simulink model "gm_soc_dvbs2_fpga"  (R2025b)
settings: Solver=VariableStepAuto  StartTime=0.0  StopTime=10.0  RelTol=1e-3
InitFcn:
  | soc_dvbs2_init;
undefined symbols (not defined in the file or in its folder): Add, coefficientsLog, coefficientsSqrt1, coefficientsSqrt2, dataBits, Deinterleaver, designMultirateFIR, noisePow, Shift, Short, soc_dvbs2_designFIRFilter, soc_dvbs2_txPacketBits, syncWord, txDataOut, txFiltCoeff, XData
libraries: simulink x304, hdlsllib x265, dspsigops x15, dsphdlfiltering2 x8, hdlmdlgenlib x6, dsphdlsigops2 x5, commseqgen3 x5, dsphdlmathfun2 x3, hwlogicconnlib x2, whdledac x2, commhdlcrc x2, whdlutilities x1
(part 25 of 36)

== system gm_soc_dvbs2_fpga/DVBS2/DVBS2 TxRx/Channel/AWGN Generator/Unit Variance Gaussian Noise/logImplementation/log/RangeReconstruction ==
  y_e : Inport  OutDataTypeStr=fixdt(1, 31, 27)  PortDimensions=1  SampleTime=6.25e-08
  exp_e : Inport  Port=2  OutDataTypeStr=uint8  PortDimensions=1  SampleTime=6.25e-08
  Add1 : Sum  Inputs=+-  OutDataTypeStr=fixdt(0, 31, 24)  AccumDataTypeStr=fixdt(1, 36, 28)  SampleTime=6.25e-08
  Bit Shift : hdlsllib/Logic and Bit Operations/Bit Shift  mode=Shift Left Logical  N=double(1)
  Constant : Constant  Value=0.69314718060195446014404296875  OutDataTypeStr=fixdt(1, 33, 32)  SampleTime=6.25e-08
  Delay{1..6} (6 alike) : Delay  DelayLength=double(2)  InitialCondition=0  SampleTime=6.25e-08
  Product : Product  Inputs=**  OutDataTypeStr=fixdt(1, 41, 32)  SampleTime=6.25e-08
  Product_out_dtc : DataTypeConversion  OutDataTypeStr=fixdt(1, 35, 28)  SampleTime=6.25e-08  SaturateOnIntegerOverflow=off  RndMeth=Floor
  e : Outport  SampleTime=6.25e-08
  wires:
  Delay1/1 -> Delay5/1
  Delay5/1 -> Add1/2
  y_e/1 -> Delay1/1
  Delay2/1 -> Product/2
  Delay3/1 -> Product/1
  Constant/1 -> Delay2/1
  exp_e/1 -> Delay3/1
  Product_out_dtc/1 -> Delay4/1
  Product/1 -> Product_out_dtc/1
  Delay4/1 -> Add1/1
  Delay6/1 -> Bit Shift/1
  Add1/1 -> Delay6/1
  Bit Shift/1 -> e/1

== system gm_soc_dvbs2_fpga/DVBS2/DVBS2 TxRx/Channel/AWGN Generator/Unit Variance Gaussian Noise/logImplementation/log/RangeReduction ==
  note: Range of x_e=[1,2)
  x : Inport  OutDataTypeStr=fixdt(0, 48, 48)  PortDimensions=1  SampleTime=6.25e-08
  Add : Sum  OutDataTypeStr=fixdt(0,49,48)
  Constant : Constant  OutDataTypeStr=uint8  SampleTime=-1
  Delay : Delay
  Delay{1,3..7} (6 alike) : Delay  DelayLength=1
  Delay2 : Delay
  Shift Arithmetic3 : ArithShift  BitShiftNumberSource=Input port  BitShiftNumber=8  BitShiftDirection=Left
      settings: InputPortMap=u0,p1
  leadingZeroDetector : MATLAB Function  TreatAsAtomicUnit=on
  x_e : Outport  SampleTime=6.25e-08
  exp_e : Outport  Port=2  SampleTime=6.25e-08  VectorParamsAs1DForOutWhenUnconnected=off
  wires:
  x/1 -> Delay3/1, Delay1/1
  leadingZeroDetector/1(exp_e) -> Delay2/1  "exp_e-1"
  Delay5/1 -> Delay7/1
  Delay2/1 -> Shift Arithmetic3/2, Delay5/1
  Delay/1 -> Shift Arithmetic3/1
  Delay3/1 -> Delay/1
  Delay1/1 -> leadingZeroDetector/1(x)
  Shift Arithmetic3/1 -> Delay4/1
  Delay4/1 -> Add/1
  Delay7/1 -> exp_e/1
  Constant/1 -> Add/2
  Add/1 -> Delay6/1
  Delay6/1 -> x_e/1

== system gm_soc_dvbs2_fpga/DVBS2/DVBS2 TxRx/DVB-S2 HDL Receiver/Demod Deinterleave and FECDecode/DVBS2 HDL Deinterleaver/RAM Address Generator/Generate and Add Read Base Address/Indicate End of Every ShortFrame Length Samples ==
  readAddr : Inport  OutDataTypeStr=fixdt(0, 17, 0)  PortDimensions=1  SampleTime=7.8125e-09
  Compare To Constant : simulink/Logic and Bit Operations/Compare To Constant  relop===  const=ConfigRx.ShortFrameLen - 1  OutDataTypeStr=boolean
  Compare To Constant1 : simulink/Logic and Bit Operations/Compare To Constant  relop===  const=ConfigRx.ShortFrameLen*2 - 1  OutDataTypeStr=boolean
  Compare To Constant2 : simulink/Logic and Bit Operations/Compare To Constant  relop===  const=ConfigRx.ShortFrameLen*3 - 1  OutDataTypeStr=boolean
  Compare To Constant3 : simulink/Logic and Bit Operations/Compare To Constant  relop===  const=ConfigRx.ShortFrameLen*4 - 1  OutDataTypeStr=boolean
  Logical Operator1 : Logic  Operator=OR  Inputs=4  AllPortsSameDT=off  OutDataTypeStr=boolean
  endIndicate : Outport  SampleTime=7.8125e-09
  wires:
  Compare To Constant/1 -> Logical Operator1/1
  readAddr/1 -> Compare To Constant3/1, Compare To Constant1/1, Compare To Constant2/1, Compare To Constant/1
  Compare To Constant2/1 -> Logical Operator1/3
  Compare To Constant1/1 -> Logical Operator1/2
  Logical Operator1/1 -> endIndicate/1
  Compare To Constant3/1 -> Logical Operator1/4

== system gm_soc_dvbs2_fpga/DVBS2/DVBS2 TxRx/DVB-S2 HDL Receiver/Demod Deinterleave and FECDecode/DVBS2 HDL Deinterleaver/RAM Address Generator/Read Offset Address/Compute Read Offset Address ==
  curR : Inport  OutDataTypeStr=uint16  PortDimensions=1  SampleTime=7.8125e-09
  maxC : Inport  Port=2  OutDataTypeStr=fixdt(0, 3, 0)  PortDimensions=1  SampleTime=7.8125e-09
  curC : Inport  Port=3  OutDataTypeStr=fixdt(0, 3, 0)  PortDimensions=1  SampleTime=7.8125e-09
  Add : Sum  OutDataTypeStr=fixdt(0, 17, 0)
  Delay1 : Delay  DelayLength=1
  Delay2 : Delay
  Delay3 : Delay
  Delay4 : Delay  DelayLength=1
  Delay5 : Delay  DelayLength=1
  Delay8 : Delay
  Product : Product  OutDataTypeStr=fixdt('ufix17')
  addr : Outport  SampleTime=7.8125e-09
  wires:
  Delay1/1 -> Add/1
  Delay3/1 -> Delay4/1
  Delay2/1 -> Product/2
  Delay5/1 -> addr/1
  maxC/1 -> Delay2/1
  curR/1 -> Delay8/1
  Product/1 -> Delay1/1
  Add/1 -> Delay5/1
  Delay8/1 -> Product/1
  curC/1 -> Delay3/1
  Delay4/1 -> Add/2

== system gm_soc_dvbs2_fpga/DVBS2/DVBS2 TxRx/DVB-S2 HDL Receiver/Demod Deinterleave and FECDecode/DVBS2 HDL Deinterleaver/RAM Address Generator/Read Offset Address/Generate Signal for End of Frame ==
  maxR : Inport  OutDataTypeStr=uint16  PortDimensions=1  SampleTime=7.8125e-09
  maxC : Inport  Port=2  OutDataTypeStr=fixdt(0, 3, 0)  PortDimensions=1  SampleTime=7.8125e-09
  Add : Sum  Inputs=+-  OutDataTypeStr=uint16
  Compare To Constant : simulink/Logic and Bit Operations/Compare To Constant  relop=~=  const=0  OutDataTypeStr=boolean
  Constant : Constant  OutDataTypeStr=fixdt('ufix1')  SampleTime=Tsamp
  Constant1 : Constant  Value=0  OutDataTypeStr=fixdt('ufix1')  SampleTime=Tsamp
  Delay : Delay
  Delay1 : Delay
  Delay2 : Delay  DelayLength=1
  Delay4 : Delay  DelayLength=1
  Product : Product  OutDataTypeStr=uint16
  Switch : Switch  Criteria=u2 > Threshold  OutDataTypeStr=fixdt(0, 1, 0)  SaturateOnIntegerOverflow=off  InputSameDT=off
  chkwrAddrEnd : Outport  SampleTime=7.8125e-09
  wires:
  Constant/1 -> Switch/1
  Delay2/1 -> Add/1, Compare To Constant/1
  Constant1/1 -> Switch/3
  Product/1 -> Delay2/1
  Delay1/1 -> Product/2
  maxR/1 -> Delay/1
  Delay/1 -> Product/1
  maxC/1 -> Delay1/1
  Switch/1 -> Add/2
  Compare To Constant/1 -> Switch/2
  Delay4/1 -> chkwrAddrEnd/1
  Add/1 -> Delay4/1

== system gm_soc_dvbs2_fpga/DVBS2/DVBS2 TxRx/DVB-S2 HDL Receiver/Demod Deinterleave and FECDecode/DVBS2 HDL Deinterleaver/RAM Address Generator/Read Offset Address/Read Offset Address Signals Generator ==
  maxR : Inport  OutDataTypeStr=uint16  PortDimensions=1  SampleTime=7.8125e-09
  chkwrAddrEnd : Inport  Port=2  OutDataTypeStr=uint16  PortDimensions=1  SampleTime=7.8125e-09
  maxC : Inport  Port=3  OutDataTypeStr=fixdt(0, 3, 0)  PortDimensions=1  SampleTime=7.8125e-09
  modcodIs12 : Inport  Port=4  OutDataTypeStr=boolean  PortDimensions=1  SampleTime=7.8125e-09
  wrAddr : Inport  Port=5  OutDataTypeStr=uint16  PortDimensions=1  SampleTime=7.8125e-09
  wrEnb : Inport  Port=6  OutDataTypeStr=boolean  PortDimensions=1  SampleTime=7.8125e-09
  Read Offset Address Signals Generator : MATLAB Function  TreatAsAtomicUnit=on  mask{isInterleave=0}
  Read Offset Address Signals Generator_term3 : Terminator
  t : Constant  Value=double(0)  OutDataTypeStr=boolean  SampleTime=7.8125e-09
  curCorROut : Outport  SampleTime=7.8125e-09  VectorParamsAs1DForOutWhenUnconnected=off
  maxRorCOut : Outport  Port=2  SampleTime=7.8125e-09
  curRorCOut : Outport  Port=3  SampleTime=7.8125e-09
  modcodIs12Out : Outport  Port=4  SampleTime=7.8125e-09
  startOut : Outport  Port=5  SampleTime=7.8125e-09
  endOut : Outport  Port=6  SampleTime=7.8125e-09
  readValid : Outport  Port=7  SampleTime=7.8125e-09
  wires:
  t/1 -> modcodIs12Out/1
  maxR/1 -> Read Offset Address Signals Generator/1(maxR)
  wrEnb/1 -> Read Offset Address Signals Generator/6(wrEnb)
  modcodIs12/1 -> Read Offset Address Signals Generator/4(modcodIs12)
  maxC/1 -> Read Offset Address Signals Generator/3(maxC)
  chkwrAddrEnd/1 -> Read Offset Address Signals Generator/2(chkwrAddrEnd)
  wrAddr/1 -> Read Offset Address Signals Generator/5(wrAddr)
  Read Offset Address Signals Generator/1(curCorROut) -> curCorROut/1
  Read Offset Address Signals Generator/2(maxRorCOut) -> maxRorCOut/1
  Read Offset Address Signals Generator/3(curRorCOut) -> curRorCOut/1
  Read Offset Address Signals Generator/4(modcodIs12Out) -> Read Offset Address Signals Generator_term3/1
  Read Offset Address Signals Generator/5(startOut) -> startOut/1
  Read Offset Address Signals Generator/6(endOut) -> endOut/1
  Read Offset Address Signals Generator/7(readValid) -> readValid/1

== system gm_soc_dvbs2_fpga/DVBS2/DVBS2 TxRx/DVB-S2 HDL Receiver/Stream Recovery/BB Decoder/Extract Stream/Extract User Packet /Indicate SYNCD bit ==
  rst : Inport  OutDataTypeStr=boolean  PortDimensions=1  SampleTime=7.8125e-09
  Distance : Inport  Port=2  OutDataTypeStr=uint16  PortDimensions=1  SampleTime=7.8125e-09
  validIn : Inport  Port=3  OutDataTypeStr=boolean  PortDimensions=1  SampleTime=7.8125e-09
  Constant1 : Constant  OutDataTypeStr=fixdt(0,1,0)  SampleTime=-1
  Constant2 : Constant  Value=0  OutDataTypeStr=fixdt(0,1,0)  SampleTime=-1
  HDL Counter1 : hdlsllib/Sources/HDL Counter  CountType=Free running  CountInit=0  CountStep=1  CountMax=25  CountFromType=Initial value  CountFrom=0  CountResetPort=on  CountLoadPort=off  CountEnbPort=on  CountDirPort=off  CountHitOutputPort=off  CountDataType=Unsigned  CountWordLen=16  CountFracLen=0  CountSampTime=1
  Logical Operator3 : Logic  AllPortsSameDT=off  OutDataTypeStr=boolean
  Relational Operator1 : RelationalOperator  Operator===  OutDataTypeStr=boolean  RndMeth=Simplest  InputSameDT=off
  Subtract1 : Sum  Inputs=+-  OutDataTypeStr=uint16
  Switch : Switch  Criteria=u2 ~= 0  OutDataTypeStr=fixdt(0, 1, 0)  SaturateOnIntegerOverflow=off  InputSameDT=off
  trigger : Outport  SampleTime=7.8125e-09
  wires:
  HDL Counter1/1 -> Relational Operator1/2
  validIn/1 -> HDL Counter1/2, Logical Operator3/2
  rst/1 -> HDL Counter1/1
  Constant2/1 -> Switch/3
  Constant1/1 -> Switch/1
  Distance/1 -> Subtract1/1, Switch/2
  Switch/1 -> Subtract1/2
  Subtract1/1 -> Relational Operator1/1
  Relational Operator1/1 -> Logical Operator3/1
  Logical Operator3/1 -> trigger/1

== system gm_soc_dvbs2_fpga/DVBS2/DVBS2 TxRx/DVB-S2 HDL Receiver/Stream Recovery/BB Decoder/Extract Stream/Extract User Packet /Sample Discard Control ==
  dataIn : Inport  OutDataTypeStr=boolean  PortDimensions=[2]  SampleTime=7.8125e-09
  startIn : Inport  Port=2  OutDataTypeStr=boolean  PortDimensions=1  SampleTime=7.8125e-09
  endIn : Inport  Port=3  OutDataTypeStr=boolean  PortDimensions=1  SampleTime=7.8125e-09
  validIn : Inport  Port=4  OutDataTypeStr=boolean  PortDimensions=1  SampleTime=7.8125e-09
  Sample Discard Control : MATLAB Function  TreatAsAtomicUnit=on
  Sample Discard Control_term1 : Terminator
  t : Constant  Value=double(0)  OutDataTypeStr=boolean  SampleTime=7.8125e-09
  dataOut : Outport  SampleTime=7.8125e-09
  startOut : Outport  Port=2  SampleTime=7.8125e-09
  endOut : Outport  Port=3  SampleTime=7.8125e-09
  validOut : Outport  Port=4  SampleTime=7.8125e-09
  wires:
  t/1 -> startOut/1
  endIn/1 -> Sample Discard Control/3(endIn)
  dataIn/1 -> Sample Discard Control/1(dataIn)
  validIn/1 -> Sample Discard Control/4(validIn)
  startIn/1 -> Sample Discard Control/2(startIn)
  Sample Discard Control/3(endOut) -> endOut/1
  Sample Discard Control/1(dataOut) -> dataOut/1
  Sample Discard Control/2(startOut) -> Sample Discard Control_term1/1
  Sample Discard Control/4(validOut) -> validOut/1

== system gm_soc_dvbs2_fpga/DVBS2/DVBS2 TxRx/DVB-S2 HDL Receiver/Stream Recovery/BB Decoder/Extract Stream/Extract User Packet /Variable Count Limited HDL Counter ==
  rst : Inport  OutDataTypeStr=boolean  PortDimensions=1  SampleTime=7.8125e-09
  countToValue : Inport  Port=2  OutDataTypeStr=uint16  PortDimensions=1  SampleTime=7.8125e-09
  enb : Inport  Port=3  OutDataTypeStr=boolean  PortDimensions=1  SampleTime=7.8125e-09
  Variable Count Limited HDL Counter : MATLAB Function  TreatAsAtomicUnit=on
  Hit : Outport  SampleTime=7.8125e-09
  wires:
  enb/1 -> Variable Count Limited HDL Counter/3(enb)
  rst/1 -> Variable Count Limited HDL Counter/1(rst)
  countToValue/1 -> Variable Count Limited HDL Counter/2(countToValue)
  Variable Count Limited HDL Counter/1(Hit) -> Hit/1

== system gm_soc_dvbs2_fpga/DVBS2/DVBS2 TxRx/DVB-S2 HDL Receiver/Synchronizer and PL Header Decoder/PL Header Recovery/PL Header Decoder/ML Decoder/Compute Euclidean Distance ==
  softBit : Inport  OutDataTypeStr=fixdt(1, 18, 13)  PortDimensions=1  SampleTime=2.5e-07
  Add : Subsystem
  Add1 : Sum  Inputs=+++  OutDataTypeStr=fixdt(1, 20, 13)
  Constant : Constant  OutDataTypeStr=fixdt(0,1,0)  SampleTime=-1
  Data Type Conversion : DataTypeConversion  OutDataTypeStr=fixdt(1, 20, 13)  SaturateOnIntegerOverflow=off  RndMeth=Floor
  Delay{1..7} (7 alike) : Delay
  Divide by 2 : DataTypeConversion  OutDataTypeStr=fixdt(1,18,12)  ConvertRealWorld=Stored Integer (SI)  SaturateOnIntegerOverflow=off  RndMeth=Floor
  Product : Product  OutDataTypeStr=fixdt(1, 18, 13)
  forBit0 : Outport  SampleTime=2.5e-07
  forBit1 : Outport  Port=2  SampleTime=2.5e-07
  wires:
  Delay3/1 -> Add1/3, Add/1(In1)
  Delay5/1 -> Delay6/1
  Delay1/1 -> Product/1
  softBit/1 -> Delay2/1, Delay1/1, Divide by 2/1
  Delay4/1 -> Delay7/1
  Delay2/1 -> Product/2
  Divide by 2/1 -> Delay5/1, Delay4/1
  Product/1 -> Delay3/1
  Constant/1 -> Add1/1, Add/3(In3)
  Delay7/1 -> Add/2(In2)
  Delay6/1 -> Add1/2
  Add/1(Out1) -> Data Type Conversion/1
  Add1/1 -> forBit0/1
  Data Type Conversion/1 -> forBit1/1

== system gm_soc_dvbs2_fpga/DVBS2/DVBS2 TxRx/DVB-S2 HDL Receiver/Synchronizer and PL Header Decoder/PL Header Recovery/PL Header Decoder/ML Decoder/Euclidean Distance Sum Up_instance1 ==
  note: For Each
  Ed0 : Inport  OutDataTypeStr=fixdt(1, 25, 15)  PortDimensions=1  SampleTime=2.5e-07
  Ed1 : Inport  Port=2  OutDataTypeStr=fixdt(1, 20, 13)  PortDimensions=1  SampleTime=2.5e-07
  reset : Inport  Port=3  OutDataTypeStr=boolean  PortDimensions=1  SampleTime=2.5e-07
  CWswitch : Inport  Port=4  OutDataTypeStr=fixdt(0, 1, 0)  PortDimensions=1  SampleTime=2.5e-07
  validIn : Inport  Port=5  OutDataTypeStr=boolean  PortDimensions=1  SampleTime=2.5e-07
  Add : Sum  OutDataTypeStr=fixdt(1, 25, 15)  AccumDataTypeStr=fixdt(1, 26, 15)  SampleTime=2.5e-07
  Delay{1..4} (4 alike) : Delay  DelayLength=double(1)  InitialCondition=0  SampleTime=2.5e-07
  Switch : Switch  Criteria=u2 ~= 0  Threshold="fi(0,0,1,0,\"hex\",\"0\")"  OutDataTypeStr=fixdt(1, 25, 15)  SampleTime=2.5e-07  SaturateOnIntegerOverflow=off  InputSameDT=off
  Unit Delay Enabled Resettable Synchronous : hdlsllib/Discrete/Unit Delay Enabled Resettable Synchronous  InitialCondition=double(0)  SampleTime=-1
  CwEdMetric : Outport  SampleTime=2.5e-07
  wires:
  Ed0/1 -> Switch/3
  reset/1 -> Delay2/1
  validIn/1 -> Delay1/1
  CWswitch/1 -> Switch/2
  Ed1/1 -> Switch/1
  Switch/1 -> Delay3/1
  Delay1/1 -> Unit Delay Enabled Resettable Synchronous/2
  Delay2/1 -> Unit Delay Enabled Resettable Synchronous/3
  Unit Delay Enabled Resettable Synchronous/1 -> Delay4/1, Add/1
  Delay3/1 -> Add/2
  Delay4/1 -> CwEdMetric/1
  Add/1 -> Unit Delay Enabled Resettable Synchronous/1

== system gm_soc_dvbs2_fpga/DVBS2/DVBS2 TxRx/DVB-S2 HDL Receiver/Synchronizer and PL Header Decoder/PL Header Recovery/PL Header Decoder/ML Decoder/Euclidean Distance Sum Up_instance10 ==
  note: For Each
  Ed0 : Inport  OutDataTypeStr=fixdt(1, 25, 15)  PortDimensions=1  SampleTime=2.5e-07
  Ed1 : Inport  Port=2  OutDataTypeStr=fixdt(1, 20, 13)  PortDimensions=1  SampleTime=2.5e-07
  reset : Inport  Port=3  OutDataTypeStr=boolean  PortDimensions=1  SampleTime=2.5e-07
  CWswitch : Inport  Port=4  OutDataTypeStr=fixdt(0, 1, 0)  PortDimensions=1  SampleTime=2.5e-07
  validIn : Inport  Port=5  OutDataTypeStr=boolean  PortDimensions=1  SampleTime=2.5e-07
  Add : Sum  OutDataTypeStr=fixdt(1, 25, 15)  AccumDataTypeStr=fixdt(1, 26, 15)  SampleTime=2.5e-07
  Delay{1..4} (4 alike) : Delay  DelayLength=double(1)  InitialCondition=0  SampleTime=2.5e-07
  Switch : Switch  Criteria=u2 ~= 0  Threshold="fi(0,0,1,0,\"hex\",\"0\")"  OutDataTypeStr=fixdt(1, 25, 15)  SampleTime=2.5e-07  SaturateOnIntegerOverflow=off  InputSameDT=off
  Unit Delay Enabled Resettable Synchronous : hdlsllib/Discrete/Unit Delay Enabled Resettable Synchronous  InitialCondition=double(0)  SampleTime=-1
  CwEdMetric : Outport  SampleTime=2.5e-07
  wires:
  Switch/1 -> Delay3/1
  validIn/1 -> Delay1/1
  Delay1/1 -> Unit Delay Enabled Resettable Synchronous/2
  reset/1 -> Delay2/1
  Delay2/1 -> Unit Delay Enabled Resettable Synchronous/3
  CWswitch/1 -> Switch/2
  Ed1/1 -> Switch/1
  Ed0/1 -> Switch/3
  Unit Delay Enabled Resettable Synchronous/1 -> Delay4/1, Add/1
  Add/1 -> Unit Delay Enabled Resettable Synchronous/1
  Delay3/1 -> Add/2
  Delay4/1 -> CwEdMetric/1

== system gm_soc_dvbs2_fpga/DVBS2/DVBS2 TxRx/DVB-S2 HDL Receiver/Synchronizer and PL Header Decoder/PL Header Recovery/PL Header Decoder/ML Decoder/Euclidean Distance Sum Up_instance11 ==
  note: For Each
  Ed0 : Inport  OutDataTypeStr=fixdt(1, 25, 15)  PortDimensions=1  SampleTime=2.5e-07
  Ed1 : Inport  Port=2  OutDataTypeStr=fixdt(1, 20, 13)  PortDimensions=1  SampleTime=2.5e-07
  reset : Inport  Port=3  OutDataTypeStr=boolean  PortDimensions=1  SampleTime=2.5e-07
  CWswitch : Inport  Port=4  OutDataTypeStr=fixdt(0, 1, 0)  PortDimensions=1  SampleTime=2.5e-07
  validIn : Inport  Port=5  OutDataTypeStr=boolean  PortDimensions=1  SampleTime=2.5e-07
  Add : Sum  OutDataTypeStr=fixdt(1, 25, 15)  AccumDataTypeStr=fixdt(1, 26, 15)  SampleTime=2.5e-07
  Delay{1..4} (4 alike) : Delay  DelayLength=double(1)  InitialCondition=0  SampleTime=2.5e-07
  Switch : Switch  Criteria=u2 ~= 0  Threshold="fi(0,0,1,0,\"hex\",\"0\")"  OutDataTypeStr=fixdt(1, 25, 15)  SampleTime=2.5e-07  SaturateOnIntegerOverflow=off  InputSameDT=off
  Unit Delay Enabled Resettable Synchronous : hdlsllib/Discrete/Unit Delay Enabled Resettable Synchronous  InitialCondition=double(0)  SampleTime=-1
  CwEdMetric : Outport  SampleTime=2.5e-07
  wires:
  Ed0/1 -> Switch/3
  reset/1 -> Delay2/1
  validIn/1 -> Delay1/1
  CWswitch/1 -> Switch/2
  Ed1/1 -> Switch/1
  Switch/1 -> Delay3/1
  Delay1/1 -> Unit Delay Enabled Resettable Synchronous/2
  Delay2/1 -> Unit Delay Enabled Resettable Synchronous/3
  Unit Delay Enabled Resettable Synchronous/1 -> Delay4/1, Add/1
  Add/1 -> Unit Delay Enabled Resettable Synchronous/1
  Delay3/1 -> Add/2
  Delay4/1 -> CwEdMetric/1

== system gm_soc_dvbs2_fpga/DVBS2/DVBS2 TxRx/DVB-S2 HDL Receiver/Synchronizer and PL Header Decoder/PL Header Recovery/PL Header Decoder/ML Decoder/Euclidean Distance Sum Up_instance12 ==
  note: For Each
  Ed0 : Inport  OutDataTypeStr=fixdt(1, 25, 15)  PortDimensions=1  SampleTime=2.5e-07
  Ed1 : Inport  Port=2  OutDataTypeStr=fixdt(1, 20, 13)  PortDimensions=1  SampleTime=2.5e-07
  reset : Inport  Port=3  OutDataTypeStr=boolean  PortDimensions=1  SampleTime=2.5e-07
  CWswitch : Inport  Port=4  OutDataTypeStr=fixdt(0, 1, 0)  PortDimensions=1  SampleTime=2.5e-07
  validIn : Inport  Port=5  OutDataTypeStr=boolean  PortDimensions=1  SampleTime=2.5e-07
  Add : Sum  OutDataTypeStr=fixdt(1, 25, 15)  AccumDataTypeStr=fixdt(1, 26, 15)  SampleTime=2.5e-07
  Delay{1..4} (4 alike) : Delay  DelayLength=double(1)  InitialCondition=0  SampleTime=2.5e-07
  Switch : Switch  Criteria=u2 ~= 0  Threshold="fi(0,0,1,0,\"hex\",\"0\")"  OutDataTypeStr=fixdt(1, 25, 15)  SampleTime=2.5e-07  SaturateOnIntegerOverflow=off  InputSameDT=off
  Unit Delay Enabled Resettable Synchronous : hdlsllib/Discrete/Unit Delay Enabled Resettable Synchronous  InitialCondition=double(0)  SampleTime=-1
  CwEdMetric : Outport  SampleTime=2.5e-07
  wires:
  Switch/1 -> Delay3/1
  validIn/1 -> Delay1/1
  Delay1/1 -> Unit Delay Enabled Resettable Synchronous/2
  reset/1 -> Delay2/1
  Delay2/1 -> Unit Delay Enabled Resettable Synchronous/3
  CWswitch/1 -> Switch/2
  Ed1/1 -> Switch/1
  Ed0/1 -> Switch/3
  Unit Delay Enabled Resettable Synchronous/1 -> Delay4/1, Add/1
  Add/1 -> Unit Delay Enabled Resettable Synchronous/1
  Delay3/1 -> Add/2
  Delay4/1 -> CwEdMetric/1

== system gm_soc_dvbs2_fpga/DVBS2/DVBS2 TxRx/DVB-S2 HDL Receiver/Synchronizer and PL Header Decoder/PL Header Recovery/PL Header Decoder/ML Decoder/Euclidean Distance Sum Up_instance13 ==
  note: For Each
  Ed0 : Inport  OutDataTypeStr=fixdt(1, 25, 15)  PortDimensions=1  SampleTime=2.5e-07
  Ed1 : Inport  Port=2  OutDataTypeStr=fixdt(1, 20, 13)  PortDimensions=1  SampleTime=2.5e-07
  reset : Inport  Port=3  OutDataTypeStr=boolean  PortDimensions=1  SampleTime=2.5e-07
  CWswitch : Inport  Port=4  OutDataTypeStr=fixdt(0, 1, 0)  PortDimensions=1  SampleTime=2.5e-07
  validIn : Inport  Port=5  OutDataTypeStr=boolean  PortDimensions=1  SampleTime=2.5e-07
  Add : Sum  OutDataTypeStr=fixdt(1, 25, 15)  AccumDataTypeStr=fixdt(1, 26, 15)  SampleTime=2.5e-07
  Delay{1..4} (4 alike) : Delay  DelayLength=double(1)  InitialCondition=0  SampleTime=2.5e-07
  Switch : Switch  Criteria=u2 ~= 0  Threshold="fi(0,0,1,0,\"hex\",\"0\")"  OutDataTypeStr=fixdt(1, 25, 15)  SampleTime=2.5e-07  SaturateOnIntegerOverflow=off  InputSameDT=off
  Unit Delay Enabled Resettable Synchronous : hdlsllib/Discrete/Unit Delay Enabled Resettable Synchronous  InitialCondition=double(0)  SampleTime=-1
  CwEdMetric : Outport  SampleTime=2.5e-07
  wires:
  Ed0/1 -> Switch/3
  reset/1 -> Delay2/1
  validIn/1 -> Delay1/1
  CWswitch/1 -> Switch/2
  Ed1/1 -> Switch/1
  Switch/1 -> Delay3/1
  Delay1/1 -> Unit Delay Enabled Resettable Synchronous/2
  Delay2/1 -> Unit Delay Enabled Resettable Synchronous/3
  Unit Delay Enabled Resettable Synchronous/1 -> Delay4/1, Add/1
  Add/1 -> Unit Delay Enabled Resettable Synchronous/1
  Delay3/1 -> Add/2
  Delay4/1 -> CwEdMetric/1

== system gm_soc_dvbs2_fpga/DVBS2/DVBS2 TxRx/DVB-S2 HDL Receiver/Synchronizer and PL Header Decoder/PL Header Recovery/PL Header Decoder/ML Decoder/Euclidean Distance Sum Up_instance14 ==
  note: For Each
  Ed0 : Inport  OutDataTypeStr=fixdt(1, 25, 15)  PortDimensions=1  SampleTime=2.5e-07
  Ed1 : Inport  Port=2  OutDataTypeStr=fixdt(1, 20, 13)  PortDimensions=1  SampleTime=2.5e-07
  reset : Inport  Port=3  OutDataTypeStr=boolean  PortDimensions=1  SampleTime=2.5e-07
  CWswitch : Inport  Port=4  OutDataTypeStr=fixdt(0, 1, 0)  PortDimensions=1  SampleTime=2.5e-07
  validIn : Inport  Port=5  OutDataTypeStr=boolean  PortDimensions=1  SampleTime=2.5e-07
  Add : Sum  OutDataTypeStr=fixdt(1, 25, 15)  AccumDataTypeStr=fixdt(1, 26, 15)  SampleTime=2.5e-07
  Delay{1..4} (4 alike) : Delay  DelayLength=double(1)  InitialCondition=0  SampleTime=2.5e-07
  Switch : Switch  Criteria=u2 ~= 0  Threshold="fi(0,0,1,0,\"hex\",\"0\")"  OutDataTypeStr=fixdt(1, 25, 15)  SampleTime=2.5e-07  SaturateOnIntegerOverflow=off  InputSameDT=off
  Unit Delay Enabled Resettable Synchronous : hdlsllib/Discrete/Unit Delay Enabled Resettable Synchronous  InitialCondition=double(0)  SampleTime=-1
  CwEdMetric : Outport  SampleTime=2.5e-07
  wires:
  Switch/1 -> Delay3/1
  validIn/1 -> Delay1/1
  Delay1/1 -> Unit Delay Enabled Resettable Synchronous/2
  reset/1 -> Delay2/1
  Ed1/1 -> Switch/1
  Delay2/1 -> Unit Delay Enabled Resettable Synchronous/3
  CWswitch/1 -> Switch/2
  Ed0/1 -> Switch/3
  Unit Delay Enabled Resettable Synchronous/1 -> Delay4/1, Add/1
  Add/1 -> Unit Delay Enabled Resettable Synchronous/1
  Delay3/1 -> Add/2
  Delay4/1 -> CwEdMetric/1

== system gm_soc_dvbs2_fpga/DVBS2/DVBS2 TxRx/DVB-S2 HDL Receiver/Synchronizer and PL Header Decoder/PL Header Recovery/PL Header Decoder/ML Decoder/Euclidean Distance Sum Up_instance15 ==
  note: For Each
  Ed0 : Inport  OutDataTypeStr=fixdt(1, 25, 15)  PortDimensions=1  SampleTime=2.5e-07
  Ed1 : Inport  Port=2  OutDataTypeStr=fixdt(1, 20, 13)  PortDimensions=1  SampleTime=2.5e-07
  reset : Inport  Port=3  OutDataTypeStr=boolean  PortDimensions=1  SampleTime=2.5e-07
  CWswitch : Inport  Port=4  OutDataTypeStr=fixdt(0, 1, 0)  PortDimensions=1  SampleTime=2.5e-07
  validIn : Inport  Port=5  OutDataTypeStr=boolean  PortDimensions=1  SampleTime=2.5e-07
  Add : Sum  OutDataTypeStr=fixdt(1, 25, 15)  AccumDataTypeStr=fixdt(1, 26, 15)  SampleTime=2.5e-07
  Delay{1..4} (4 alike) : Delay  DelayLength=double(1)  InitialCondition=0  SampleTime=2.5e-07
  Switch : Switch  Criteria=u2 ~= 0  Threshold="fi(0,0,1,0,\"hex\",\"0\")"  OutDataTypeStr=fixdt(1, 25, 15)  SampleTime=2.5e-07  SaturateOnIntegerOverflow=off  InputSameDT=off
  Unit Delay Enabled Resettable Synchronous : hdlsllib/Discrete/Unit Delay Enabled Resettable Synchronous  InitialCondition=double(0)  SampleTime=-1
  CwEdMetric : Outport  SampleTime=2.5e-07
  wires:
  Ed0/1 -> Switch/3
  reset/1 -> Delay2/1
  validIn/1 -> Delay1/1
  CWswitch/1 -> Switch/2
  Ed1/1 -> Switch/1
  Switch/1 -> Delay3/1
  Delay1/1 -> Unit Delay Enabled Resettable Synchronous/2
  Delay2/1 -> Unit Delay Enabled Resettable Synchronous/3
  Unit Delay Enabled Resettable Synchronous/1 -> Delay4/1, Add/1
  Delay3/1 -> Add/2
  Delay4/1 -> CwEdMetric/1
  Add/1 -> Unit Delay Enabled Resettable Synchronous/1

== system gm_soc_dvbs2_fpga/DVBS2/DVBS2 TxRx/DVB-S2 HDL Receiver/Synchronizer and PL Header Decoder/PL Header Recovery/PL Header Decoder/ML Decoder/Euclidean Distance Sum Up_instance16 ==
  note: For Each
  Ed0 : Inport  OutDataTypeStr=fixdt(1, 25, 15)  PortDimensions=1  SampleTime=2.5e-07
  Ed1 : Inport  Port=2  OutDataTypeStr=fixdt(1, 20, 13)  PortDimensions=1  SampleTime=2.5e-07
  reset : Inport  Port=3  OutDataTypeStr=boolean  PortDimensions=1  SampleTime=2.5e-07
  CWswitch : Inport  Port=4  OutDataTypeStr=fixdt(0, 1, 0)  PortDimensions=1  SampleTime=2.5e-07
  validIn : Inport  Port=5  OutDataTypeStr=boolean  PortDimensions=1  SampleTime=2.5e-07
  Add : Sum  OutDataTypeStr=fixdt(1, 25, 15)  AccumDataTypeStr=fixdt(1, 26, 15)  SampleTime=2.5e-07
  Delay{1..4} (4 alike) : Delay  DelayLength=double(1)  InitialCondition=0  SampleTime=2.5e-07
  Switch : Switch  Criteria=u2 ~= 0  Threshold="fi(0,0,1,0,\"hex\",\"0\")"  OutDataTypeStr=fixdt(1, 25, 15)  SampleTime=2.5e-07  SaturateOnIntegerOverflow=off  InputSameDT=off
  Unit Delay Enabled Resettable Synchronous : hdlsllib/Discrete/Unit Delay Enabled Resettable Synchronous  InitialCondition=double(0)  SampleTime=-1
  CwEdMetric : Outport  SampleTime=2.5e-07
  wires:
  Switch/1 -> Delay3/1
  validIn/1 -> Delay1/1
  Delay1/1 -> Unit Delay Enabled Resettable Synchronous/2
  Ed0/1 -> Switch/3
  reset/1 -> Delay2/1
  Ed1/1 -> Switch/1
  Delay2/1 -> Unit Delay Enabled Resettable Synchronous/3
  CWswitch/1 -> Switch/2
  Unit Delay Enabled Resettable Synchronous/1 -> Add/1, Delay4/1
  Add/1 -> Unit Delay Enabled Resettable Synchronous/1
  Delay3/1 -> Add/2
  Delay4/1 -> CwEdMetric/1

== system gm_soc_dvbs2_fpga/DVBS2/DVBS2 TxRx/DVB-S2 HDL Receiver/Synchronizer and PL Header Decoder/PL Header Recovery/PL Header Decoder/ML Decoder/Euclidean Distance Sum Up_instance17 ==
  note: For Each
  Ed0 : Inport  OutDataTypeStr=fixdt(1, 25, 15)  PortDimensions=1  SampleTime=2.5e-07
  Ed1 : Inport  Port=2  OutDataTypeStr=fixdt(1, 20, 13)  PortDimensions=1  SampleTime=2.5e-07
  reset : Inport  Port=3  OutDataTypeStr=boolean  PortDimensions=1  SampleTime=2.5e-07
  CWswitch : Inport  Port=4  OutDataTypeStr=fixdt(0, 1, 0)  PortDimensions=1  SampleTime=2.5e-07
  validIn : Inport  Port=5  OutDataTypeStr=boolean  PortDimensions=1  SampleTime=2.5e-07
  Add : Sum  OutDataTypeStr=fixdt(1, 25, 15)  AccumDataTypeStr=fixdt(1, 26, 15)  SampleTime=2.5e-07
  Delay{1..4} (4 alike) : Delay  DelayLength=double(1)  InitialCondition=0  SampleTime=2.5e-07
  Switch : Switch  Criteria=u2 ~= 0  Threshold="fi(0,0,1,0,\"hex\",\"0\")"  OutDataTypeStr=fixdt(1, 25, 15)  SampleTime=2.5e-07  SaturateOnIntegerOverflow=off  InputSameDT=off
  Unit Delay Enabled Resettable Synchronous : hdlsllib/Discrete/Unit Delay Enabled Resettable Synchronous  InitialCondition=double(0)  SampleTime=-1
  CwEdMetric : Outport  SampleTime=2.5e-07
  wires:
  Ed0/1 -> Switch/3
  reset/1 -> Delay2/1
  validIn/1 -> Delay1/1
  Delay2/1 -> Unit Delay Enabled Resettable Synchronous/3
  CWswitch/1 -> Switch/2
  Ed1/1 -> Switch/1
  Switch/1 -> Delay3/1
  Delay1/1 -> Unit Delay Enabled Resettable Synchronous/2
  Unit Delay Enabled Resettable Synchronous/1 -> Delay4/1, Add/1
  Delay3/1 -> Add/2
  Delay4/1 -> CwEdMetric/1
  Add/1 -> Unit Delay Enabled Resettable Synchronous/1

== system gm_soc_dvbs2_fpga/DVBS2/DVBS2 TxRx/DVB-S2 HDL Receiver/Synchronizer and PL Header Decoder/PL Header Recovery/PL Header Decoder/ML Decoder/Euclidean Distance Sum Up_instance18 ==
  note: For Each
  Ed0 : Inport  OutDataTypeStr=fixdt(1, 25, 15)  PortDimensions=1  SampleTime=2.5e-07
  Ed1 : Inport  Port=2  OutDataTypeStr=fixdt(1, 20, 13)  PortDimensions=1  SampleTime=2.5e-07
  reset : Inport  Port=3  OutDataTypeStr=boolean  PortDimensions=1  SampleTime=2.5e-07
  CWswitch : Inport  Port=4  OutDataTypeStr=fixdt(0, 1, 0)  PortDimensions=1  SampleTime=2.5e-07
  validIn : Inport  Port=5  OutDataTypeStr=boolean  PortDimensions=1  SampleTime=2.5e-07
  Add : Sum  OutDataTypeStr=fixdt(1, 25, 15)  AccumDataTypeStr=fixdt(1, 26, 15)  SampleTime=2.5e-07
  Delay{1..4} (4 alike) : Delay  DelayLength=double(1)  InitialCondition=0  SampleTime=2.5e-07
  Switch : Switch  Criteria=u2 ~= 0  Threshold="fi(0,0,1,0,\"hex\",\"0\")"  OutDataTypeStr=fixdt(1, 25, 15)  SampleTime=2.5e-07  SaturateOnIntegerOverflow=off  InputSameDT=off
  Unit Delay Enabled Resettable Synchronous : hdlsllib/Discrete/Unit Delay Enabled Resettable Synchronous  InitialCondition=double(0)  SampleTime=-1
  CwEdMetric : Outport  SampleTime=2.5e-07
  wires:
  Switch/1 -> Delay3/1
  validIn/1 -> Delay1/1
  Delay1/1 -> Unit Delay Enabled Resettable Synchronous/2
  Ed0/1 -> Switch/3
  reset/1 -> Delay2/1
  Ed1/1 -> Switch/1
  Delay2/1 -> Unit Delay Enabled Resettable Synchronous/3
  CWswitch/1 -> Switch/2
  Unit Delay Enabled Resettable Synchronous/1 -> Delay4/1, Add/1
  Add/1 -> Unit Delay Enabled Resettable Synchronous/1
  Delay3/1 -> Add/2
  Delay4/1 -> CwEdMetric/1

== system gm_soc_dvbs2_fpga/DVBS2/DVBS2 TxRx/DVB-S2 HDL Receiver/Synchronizer and PL Header Decoder/PL Header Recovery/PL Header Decoder/ML Decoder/Euclidean Distance Sum Up_instance19 ==
  note: For Each
  Ed0 : Inport  OutDataTypeStr=fixdt(1, 25, 15)  PortDimensions=1  SampleTime=2.5e-07
  Ed1 : Inport  Port=2  OutDataTypeStr=fixdt(1, 20, 13)  PortDimensions=1  SampleTime=2.5e-07
  reset : Inport  Port=3  OutDataTypeStr=boolean  PortDimensions=1  SampleTime=2.5e-07
  CWswitch : Inport  Port=4  OutDataTypeStr=fixdt(0, 1, 0)  PortDimensions=1  SampleTime=2.5e-07
  validIn : Inport  Port=5  OutDataTypeStr=boolean  PortDimensions=1  SampleTime=2.5e-07
  Add : Sum  OutDataTypeStr=fixdt(1, 25, 15)  AccumDataTypeStr=fixdt(1, 26, 15)  SampleTime=2.5e-07
  Delay{1..4} (4 alike) : Delay  DelayLength=double(1)  InitialCondition=0  SampleTime=2.5e-07
  Switch : Switch  Criteria=u2 ~= 0  Threshold="fi(0,0,1,0,\"hex\",\"0\")"  OutDataTypeStr=fixdt(1, 25, 15)  SampleTime=2.5e-07  SaturateOnIntegerOverflow=off  InputSameDT=off
  Unit Delay Enabled Resettable Synchronous : hdlsllib/Discrete/Unit Delay Enabled Resettable Synchronous  InitialCondition=double(0)  SampleTime=-1
  CwEdMetric : Outport  SampleTime=2.5e-07
  wires:
  Ed0/1 -> Switch/3
  reset/1 -> Delay2/1
  validIn/1 -> Delay1/1
  Delay2/1 -> Unit Delay Enabled Resettable Synchronous/3
  CWswitch/1 -> Switch/2
  Ed1/1 -> Switch/1
  Switch/1 -> Delay3/1
  Delay1/1 -> Unit Delay Enabled Resettable Synchronous/2
  Unit Delay Enabled Resettable Synchronous/1 -> Delay4/1, Add/1
  Delay3/1 -> Add/2
  Delay4/1 -> CwEdMetric/1
  Add/1 -> Unit Delay Enabled Resettable Synchronous/1

== system gm_soc_dvbs2_fpga/DVBS2/DVBS2 TxRx/DVB-S2 HDL Receiver/Synchronizer and PL Header Decoder/PL Header Recovery/PL Header Decoder/ML Decoder/Euclidean Distance Sum Up_instance2 ==
  note: For Each
  Ed0 : Inport  OutDataTypeStr=fixdt(1, 25, 15)  PortDimensions=1  SampleTime=2.5e-07
  Ed1 : Inport  Port=2  OutDataTypeStr=fixdt(1, 20, 13)  PortDimensions=1  SampleTime=2.5e-07
  reset : Inport  Port=3  OutDataTypeStr=boolean  PortDimensions=1  SampleTime=2.5e-07
  CWswitch : Inport  Port=4  OutDataTypeStr=fixdt(0, 1, 0)  PortDimensions=1  SampleTime=2.5e-07
  validIn : Inport  Port=5  OutDataTypeStr=boolean  PortDimensions=1  SampleTime=2.5e-07
  Add : Sum  OutDataTypeStr=fixdt(1, 25, 15)  AccumDataTypeStr=fixdt(1, 26, 15)  SampleTime=2.5e-07
  Delay{1..4} (4 alike) : Delay  DelayLength=double(1)  InitialCondition=0  SampleTime=2.5e-07
  Switch : Switch  Criteria=u2 ~= 0  Threshold="fi(0,0,1,0,\"hex\",\"0\")"  OutDataTypeStr=fixdt(1, 25, 15)  SampleTime=2.5e-07  SaturateOnIntegerOverflow=off  InputSameDT=off
  Unit Delay Enabled Resettable Synchronous : hdlsllib/Discrete/Unit Delay Enabled Resettable Synchronous  InitialCondition=double(0)  SampleTime=-1
  CwEdMetric : Outport  SampleTime=2.5e-07
  wires:
  reset/1 -> Delay2/1
  validIn/1 -> Delay1/1
  Delay2/1 -> Unit Delay Enabled Resettable Synchronous/3
  Ed1/1 -> Switch/1
  CWswitch/1 -> Switch/2
  Switch/1 -> Delay3/1
  Delay1/1 -> Unit Delay Enabled Resettable Synchronous/2
  Ed0/1 -> Switch/3
  Unit Delay Enabled Resettable Synchronous/1 -> Delay4/1, Add/1
  Add/1 -> Unit Delay Enabled Resettable Synchronous/1
  Delay3/1 -> Add/2
  Delay4/1 -> CwEdMetric/1

== system gm_soc_dvbs2_fpga/DVBS2/DVBS2 TxRx/DVB-S2 HDL Receiver/Synchronizer and PL Header Decoder/PL Header Recovery/PL Header Decoder/ML Decoder/Euclidean Distance Sum Up_instance20 ==
  note: For Each
  Ed0 : Inport  OutDataTypeStr=fixdt(1, 25, 15)  PortDimensions=1  SampleTime=2.5e-07
  Ed1 : Inport  Port=2  OutDataTypeStr=fixdt(1, 20, 13)  PortDimensions=1  SampleTime=2.5e-07
  reset : Inport  Port=3  OutDataTypeStr=boolean  PortDimensions=1  SampleTime=2.5e-07
  CWswitch : Inport  Port=4  OutDataTypeStr=fixdt(0, 1, 0)  PortDimensions=1  SampleTime=2.5e-07
  validIn : Inport  Port=5  OutDataTypeStr=boolean  PortDimensions=1  SampleTime=2.5e-07
  Add : Sum  OutDataTypeStr=fixdt(1, 25, 15)  AccumDataTypeStr=fixdt(1, 26, 15)  SampleTime=2.5e-07
  Delay{1..4} (4 alike) : Delay  DelayLength=double(1)  InitialCondition=0  SampleTime=2.5e-07
  Switch : Switch  Criteria=u2 ~= 0  Threshold="fi(0,0,1,0,\"hex\",\"0\")"  OutDataTypeStr=fixdt(1, 25, 15)  SampleTime=2.5e-07  SaturateOnIntegerOverflow=off  InputSameDT=off
  Unit Delay Enabled Resettable Synchronous : hdlsllib/Discrete/Unit Delay Enabled Resettable Synchronous  InitialCondition=double(0)  SampleTime=-1
  CwEdMetric : Outport  SampleTime=2.5e-07
  wires:
  Switch/1 -> Delay3/1
  validIn/1 -> Delay1/1
  Delay1/1 -> Unit Delay Enabled Resettable Synchronous/2
  Ed0/1 -> Switch/3
  reset/1 -> Delay2/1
  CWswitch/1 -> Switch/2
  Ed1/1 -> Switch/1
  Delay2/1 -> Unit Delay Enabled Resettable Synchronous/3
  Unit Delay Enabled Resettable Synchronous/1 -> Delay4/1, Add/1
  Add/1 -> Unit Delay Enabled Resettable Synchronous/1
  Delay3/1 -> Add/2
  Delay4/1 -> CwEdMetric/1

== system gm_soc_dvbs2_fpga/DVBS2/DVBS2 TxRx/DVB-S2 HDL Receiver/Synchronizer and PL Header Decoder/PL Header Recovery/PL Header Decoder/ML Decoder/Euclidean Distance Sum Up_instance21 ==
  note: For Each
  Ed0 : Inport  OutDataTypeStr=fixdt(1, 25, 15)  PortDimensions=1  SampleTime=2.5e-07
  Ed1 : Inport  Port=2  OutDataTypeStr=fixdt(1, 20, 13)  PortDimensions=1  SampleTime=2.5e-07
  reset : Inport  Port=3  OutDataTypeStr=boolean  PortDimensions=1  SampleTime=2.5e-07
  CWswitch : Inport  Port=4  OutDataTypeStr=fixdt(0, 1, 0)  PortDimensions=1  SampleTime=2.5e-07
  validIn : Inport  Port=5  OutDataTypeStr=boolean  PortDimensions=1  SampleTime=2.5e-07
  Add : Sum  OutDataTypeStr=fixdt(1, 25, 15)  AccumDataTypeStr=fixdt(1, 26, 15)  SampleTime=2.5e-07
  Delay{1..4} (4 alike) : Delay  DelayLength=double(1)  InitialCondition=0  SampleTime=2.5e-07
  Switch : Switch  Criteria=u2 ~= 0  Threshold="fi(0,0,1,0,\"hex\",\"0\")"  OutDataTypeStr=fixdt(1, 25, 15)  SampleTime=2.5e-07  SaturateOnIntegerOverflow=off  InputSameDT=off
  Unit Delay Enabled Resettable Synchronous : hdlsllib/Discrete/Unit Delay Enabled Resettable Synchronous  InitialCondition=double(0)  SampleTime=-1
  CwEdMetric : Outport  SampleTime=2.5e-07
  wires:
  validIn/1 -> Delay1/1
  Delay1/1 -> Unit Delay Enabled Resettable Synchronous/2
  Ed0/1 -> Switch/3
  reset/1 -> Delay2/1
  Delay2/1 -> Unit Delay Enabled Resettable Synchronous/3
  CWswitch/1 -> Switch/2
  Ed1/1 -> Switch/1
  Switch/1 -> Delay3/1
  Unit Delay Enabled Resettable Synchronous/1 -> Delay4/1, Add/1
  Delay3/1 -> Add/2
  Delay4/1 -> CwEdMetric/1
  Add/1 -> Unit Delay Enabled Resettable Synchronous/1

== system gm_soc_dvbs2_fpga/DVBS2/DVBS2 TxRx/DVB-S2 HDL Receiver/Synchronizer and PL Header Decoder/PL Header Recovery/PL Header Decoder/ML Decoder/Euclidean Distance Sum Up_instance22 ==
  note: For Each
  Ed0 : Inport  OutDataTypeStr=fixdt(1, 25, 15)  PortDimensions=1  SampleTime=2.5e-07
  Ed1 : Inport  Port=2  OutDataTypeStr=fixdt(1, 20, 13)  PortDimensions=1  SampleTime=2.5e-07
  reset : Inport  Port=3  OutDataTypeStr=boolean  PortDimensions=1  SampleTime=2.5e-07
  CWswitch : Inport  Port=4  OutDataTypeStr=fixdt(0, 1, 0)  PortDimensions=1  SampleTime=2.5e-07
  validIn : Inport  Port=5  OutDataTypeStr=boolean  PortDimensions=1  SampleTime=2.5e-07
  Add : Sum  OutDataTypeStr=fixdt(1, 25, 15)  AccumDataTypeStr=fixdt(1, 26, 15)  SampleTime=2.5e-07
  Delay{1..4} (4 alike) : Delay  DelayLength=double(1)  InitialCondition=0  SampleTime=2.5e-07
  Switch : Switch  Criteria=u2 ~= 0  Threshold="fi(0,0,1,0,\"hex\",\"0\")"  OutDataTypeStr=fixdt(1, 25, 15)  SampleTime=2.5e-07  SaturateOnIntegerOverflow=off  InputSameDT=off
  Unit Delay Enabled Resettable Synchronous : hdlsllib/Discrete/Unit Delay Enabled Resettable Synchronous  InitialCondition=double(0)  SampleTime=-1
  CwEdMetric : Outport  SampleTime=2.5e-07
  wires:
  Switch/1 -> Delay3/1
  validIn/1 -> Delay1/1
  Delay1/1 -> Unit Delay Enabled Resettable Synchronous/2
  Ed0/1 -> Switch/3
  reset/1 -> Delay2/1
  CWswitch/1 -> Switch/2
  Ed1/1 -> Switch/1
  Delay2/1 -> Unit Delay Enabled Resettable Synchronous/3
  Unit Delay Enabled Resettable Synchronous/1 -> Delay4/1, Add/1
  Add/1 -> Unit Delay Enabled Resettable Synchronous/1
  Delay3/1 -> Add/2
  Delay4/1 -> CwEdMetric/1

== system gm_soc_dvbs2_fpga/DVBS2/DVBS2 TxRx/DVB-S2 HDL Receiver/Synchronizer and PL Header Decoder/PL Header Recovery/PL Header Decoder/ML Decoder/Euclidean Distance Sum Up_instance23 ==
  note: For Each
  Ed0 : Inport  OutDataTypeStr=fixdt(1, 25, 15)  PortDimensions=1  SampleTime=2.5e-07
  Ed1 : Inport  Port=2  OutDataTypeStr=fixdt(1, 20, 13)  PortDimensions=1  SampleTime=2.5e-07
  reset : Inport  Port=3  OutDataTypeStr=boolean  PortDimensions=1  SampleTime=2.5e-07
  CWswitch : Inport  Port=4  OutDataTypeStr=fixdt(0, 1, 0)  PortDimensions=1  SampleTime=2.5e-07
  validIn : Inport  Port=5  OutDataTypeStr=boolean  PortDimensions=1  SampleTime=2.5e-07
  Add : Sum  OutDataTypeStr=fixdt(1, 25, 15)  AccumDataTypeStr=fixdt(1, 26, 15)  SampleTime=2.5e-07
  Delay{1..4} (4 alike) : Delay  DelayLength=double(1)  InitialCondition=0  SampleTime=2.5e-07
  Switch : Switch  Criteria=u2 ~= 0  Threshold="fi(0,0,1,0,\"hex\",\"0\")"  OutDataTypeStr=fixdt(1, 25, 15)  SampleTime=2.5e-07  SaturateOnIntegerOverflow=off  InputSameDT=off
  Unit Delay Enabled Resettable Synchronous : hdlsllib/Discrete/Unit Delay Enabled Resettable Synchronous  InitialCondition=double(0)  SampleTime=-1
  CwEdMetric : Outport  SampleTime=2.5e-07
  wires:
  validIn/1 -> Delay1/1
  Delay1/1 -> Unit Delay Enabled Resettable Synchronous/2
  Ed0/1 -> Switch/3
  reset/1 -> Delay2/1
  Delay2/1 -> Unit Delay Enabled Resettable Synchronous/3
  CWswitch/1 -> Switch/2
  Ed1/1 -> Switch/1
  Switch/1 -> Delay3/1
  Unit Delay Enabled Resettable Synchronous/1 -> Delay4/1, Add/1
  Delay3/1 -> Add/2
  Delay4/1 -> CwEdMetric/1
  Add/1 -> Unit Delay Enabled Resettable Synchronous/1

== system gm_soc_dvbs2_fpga/DVBS2/DVBS2 TxRx/DVB-S2 HDL Receiver/Synchronizer and PL Header Decoder/PL Header Recovery/PL Header Decoder/ML Decoder/Euclidean Distance Sum Up_instance24 ==
  note: For Each
  Ed0 : Inport  OutDataTypeStr=fixdt(1, 25, 15)  PortDimensions=1  SampleTime=2.5e-07
  Ed1 : Inport  Port=2  OutDataTypeStr=fixdt(1, 20, 13)  PortDimensions=1  SampleTime=2.5e-07
  reset : Inport  Port=3  OutDataTypeStr=boolean  PortDimensions=1  SampleTime=2.5e-07
  CWswitch : Inport  Port=4  OutDataTypeStr=fixdt(0, 1, 0)  PortDimensions=1  SampleTime=2.5e-07
  validIn : Inport  Port=5  OutDataTypeStr=boolean  PortDimensions=1  SampleTime=2.5e-07
  Add : Sum  OutDataTypeStr=fixdt(1, 25, 15)  AccumDataTypeStr=fixdt(1, 26, 15)  SampleTime=2.5e-07
  Delay{1..4} (4 alike) : Delay  DelayLength=double(1)  InitialCondition=0  SampleTime=2.5e-07
  Switch : Switch  Criteria=u2 ~= 0  Threshold="fi(0,0,1,0,\"hex\",\"0\")"  OutDataTypeStr=fixdt(1, 25, 15)  SampleTime=2.5e-07  SaturateOnIntegerOverflow=off  InputSameDT=off
  Unit Delay Enabled Resettable Synchronous : hdlsllib/Discrete/Unit Delay Enabled Resettable Synchronous  InitialCondition=double(0)  SampleTime=-1
  CwEdMetric : Outport  SampleTime=2.5e-07
  wires:
  Switch/1 -> Delay3/1
  validIn/1 -> Delay1/1
  Delay1/1 -> Unit Delay Enabled Resettable Synchronous/2
  Ed0/1 -> Switch/3
  reset/1 -> Delay2/1
  CWswitch/1 -> Switch/2
  Ed1/1 -> Switch/1
  Delay2/1 -> Unit Delay Enabled Resettable Synchronous/3
  Unit Delay Enabled Resettable Synchronous/1 -> Delay4/1, Add/1
  Add/1 -> Unit Delay Enabled Resettable Synchronous/1
  Delay3/1 -> Add/2
  Delay4/1 -> CwEdMetric/1

== system gm_soc_dvbs2_fpga/DVBS2/DVBS2 TxRx/DVB-S2 HDL Receiver/Synchronizer and PL Header Decoder/PL Header Recovery/PL Header Decoder/ML Decoder/Euclidean Distance Sum Up_instance25 ==
  note: For Each
  Ed0 : Inport  OutDataTypeStr=fixdt(1, 25, 15)  PortDimensions=1  SampleTime=2.5e-07
  Ed1 : Inport  Port=2  OutDataTypeStr=fixdt(1, 20, 13)  PortDimensions=1  SampleTime=2.5e-07
  reset : Inport  Port=3  OutDataTypeStr=boolean  PortDimensions=1  SampleTime=2.5e-07
  CWswitch : Inport  Port=4  OutDataTypeStr=fixdt(0, 1, 0)  PortDimensions=1  SampleTime=2.5e-07
  validIn : Inport  Port=5  OutDataTypeStr=boolean  PortDimensions=1  SampleTime=2.5e-07
  Add : Sum  OutDataTypeStr=fixdt(1, 25, 15)  AccumDataTypeStr=fixdt(1, 26, 15)  SampleTime=2.5e-07
  Delay{1..4} (4 alike) : Delay  DelayLength=double(1)  InitialCondition=0  SampleTime=2.5e-07
  Switch : Switch  Criteria=u2 ~= 0  Threshold="fi(0,0,1,0,\"hex\",\"0\")"  OutDataTypeStr=fixdt(1, 25, 15)  SampleTime=2.5e-07  SaturateOnIntegerOverflow=off  InputSameDT=off
  Unit Delay Enabled Resettable Synchronous : hdlsllib/Discrete/Unit Delay Enabled Resettable Synchronous  InitialCondition=double(0)  SampleTime=-1
  CwEdMetric : Outport  SampleTime=2.5e-07
  wires:
  validIn/1 -> Delay1/1
  Delay1/1 -> Unit Delay Enabled Resettable Synchronous/2
  Ed0/1 -> Switch/3
  reset/1 -> Delay2/1
  Delay2/1 -> Unit Delay Enabled Resettable Synchronous/3
  CWswitch/1 -> Switch/2
  Ed1/1 -> Switch/1
  Switch/1 -> Delay3/1
  Unit Delay Enabled Resettable Synchronous/1 -> Delay4/1, Add/1
  Delay3/1 -> Add/2
  Delay4/1 -> CwEdMetric/1
  Add/1 -> Unit Delay Enabled Resettable Synchronous/1

== system gm_soc_dvbs2_fpga/DVBS2/DVBS2 TxRx/DVB-S2 HDL Receiver/Synchronizer and PL Header Decoder/PL Header Recovery/PL Header Decoder/ML Decoder/Euclidean Distance Sum Up_instance26 ==
  note: For Each
  Ed0 : Inport  OutDataTypeStr=fixdt(1, 25, 15)  PortDimensions=1  SampleTime=2.5e-07
  Ed1 : Inport  Port=2  OutDataTypeStr=fixdt(1, 20, 13)  PortDimensions=1  SampleTime=2.5e-07
  reset : Inport  Port=3  OutDataTypeStr=boolean  PortDimensions=1  SampleTime=2.5e-07
  CWswitch : Inport  Port=4  OutDataTypeStr=fixdt(0, 1, 0)  PortDimensions=1  SampleTime=2.5e-07
  validIn : Inport  Port=5  OutDataTypeStr=boolean  PortDimensions=1  SampleTime=2.5e-07
  Add : Sum  OutDataTypeStr=fixdt(1, 25, 15)  AccumDataTypeStr=fixdt(1, 26, 15)  SampleTime=2.5e-07
  Delay{1..4} (4 alike) : Delay  DelayLength=double(1)  InitialCondition=0  SampleTime=2.5e-07
  Switch : Switch  Criteria=u2 ~= 0  Threshold="fi(0,0,1,0,\"hex\",\"0\")"  OutDataTypeStr=fixdt(1, 25, 15)  SampleTime=2.5e-07  SaturateOnIntegerOverflow=off  InputSameDT=off
  Unit Delay Enabled Resettable Synchronous : hdlsllib/Discrete/Unit Delay Enabled Resettable Synchronous  InitialCondition=double(0)  SampleTime=-1
  CwEdMetric : Outport  SampleTime=2.5e-07
  wires:
  Switch/1 -> Delay3/1
  validIn/1 -> Delay1/1
  Delay1/1 -> Unit Delay Enabled Resettable Synchronous/2
  Ed0/1 -> Switch/3
  reset/1 -> Delay2/1
  CWswitch/1 -> Switch/2
  Ed1/1 -> Switch/1
  Delay2/1 -> Unit Delay Enabled Resettable Synchronous/3
  Unit Delay Enabled Resettable Synchronous/1 -> Delay4/1, Add/1
  Add/1 -> Unit Delay Enabled Resettable Synchronous/1
  Delay3/1 -> Add/2
  Delay4/1 -> CwEdMetric/1

== system gm_soc_dvbs2_fpga/DVBS2/DVBS2 TxRx/DVB-S2 HDL Receiver/Synchronizer and PL Header Decoder/PL Header Recovery/PL Header Decoder/ML Decoder/Euclidean Distance Sum Up_instance27 ==
  note: For Each
  Ed0 : Inport  OutDataTypeStr=fixdt(1, 25, 15)  PortDimensions=1  SampleTime=2.5e-07
  Ed1 : Inport  Port=2  OutDataTypeStr=fixdt(1, 20, 13)  PortDimensions=1  SampleTime=2.5e-07
  reset : Inport  Port=3  OutDataTypeStr=boolean  PortDimensions=1  SampleTime=2.5e-07
  CWswitch : Inport  Port=4  OutDataTypeStr=fixdt(0, 1, 0)  PortDimensions=1  SampleTime=2.5e-07
  validIn : Inport  Port=5  OutDataTypeStr=boolean  PortDimensions=1  SampleTime=2.5e-07
  Add : Sum  OutDataTypeStr=fixdt(1, 25, 15)  AccumDataTypeStr=fixdt(1, 26, 15)  SampleTime=2.5e-07
  Delay{1..4} (4 alike) : Delay  DelayLength=double(1)  InitialCondition=0  SampleTime=2.5e-07
  Switch : Switch  Criteria=u2 ~= 0  Threshold="fi(0,0,1,0,\"hex\",\"0\")"  OutDataTypeStr=fixdt(1, 25, 15)  SampleTime=2.5e-07  SaturateOnIntegerOverflow=off  InputSameDT=off
  Unit Delay Enabled Resettable Synchronous : hdlsllib/Discrete/Unit Delay Enabled Resettable Synchronous  InitialCondition=double(0)  SampleTime=-1
  CwEdMetric : Outport  SampleTime=2.5e-07
  wires:
  Switch/1 -> Delay3/1
  validIn/1 -> Delay1/1
  Delay1/1 -> Unit Delay Enabled Resettable Synchronous/2
  Ed0/1 -> Switch/3
  reset/1 -> Delay2/1
  Delay2/1 -> Unit Delay Enabled Resettable Synchronous/3
  CWswitch/1 -> Switch/2
  Ed1/1 -> Switch/1
  Unit Delay Enabled Resettable Synchronous/1 -> Delay4/1, Add/1
  Delay3/1 -> Add/2
  Delay4/1 -> CwEdMetric/1
  Add/1 -> Unit Delay Enabled Resettable Synchronous/1

== system gm_soc_dvbs2_fpga/DVBS2/DVBS2 TxRx/DVB-S2 HDL Receiver/Synchronizer and PL Header Decoder/PL Header Recovery/PL Header Decoder/ML Decoder/Euclidean Distance Sum Up_instance28 ==
  note: For Each
  Ed0 : Inport  OutDataTypeStr=fixdt(1, 25, 15)  PortDimensions=1  SampleTime=2.5e-07
  Ed1 : Inport  Port=2  OutDataTypeStr=fixdt(1, 20, 13)  PortDimensions=1  SampleTime=2.5e-07
  reset : Inport  Port=3  OutDataTypeStr=boolean  PortDimensions=1  SampleTime=2.5e-07
  CWswitch : Inport  Port=4  OutDataTypeStr=fixdt(0, 1, 0)  PortDimensions=1  SampleTime=2.5e-07
  validIn : Inport  Port=5  OutDataTypeStr=boolean  PortDimensions=1  SampleTime=2.5e-07
  Add : Sum  OutDataTypeStr=fixdt(1, 25, 15)  AccumDataTypeStr=fixdt(1, 26, 15)  SampleTime=2.5e-07
  Delay{1..4} (4 alike) : Delay  DelayLength=double(1)  InitialCondition=0  SampleTime=2.5e-07
  Switch : Switch  Criteria=u2 ~= 0  Threshold="fi(0,0,1,0,\"hex\",\"0\")"  OutDataTypeStr=fixdt(1, 25, 15)  SampleTime=2.5e-07  SaturateOnIntegerOverflow=off  InputSameDT=off
  Unit Delay Enabled Resettable Synchronous : hdlsllib/Discrete/Unit Delay Enabled Resettable Synchronous  InitialCondition=double(0)  SampleTime=-1
  CwEdMetric : Outport  SampleTime=2.5e-07
  wires:
  Switch/1 -> Delay3/1
  validIn/1 -> Delay1/1
  Delay1/1 -> Unit Delay Enabled Resettable Synchronous/2
  Ed0/1 -> Switch/3
  reset/1 -> Delay2/1
  CWswitch/1 -> Switch/2
  Ed1/1 -> Switch/1
  Delay2/1 -> Unit Delay Enabled Resettable Synchronous/3
  Unit Delay Enabled Resettable Synchronous/1 -> Delay4/1, Add/1
  Add/1 -> Unit Delay Enabled Resettable Synchronous/1
  Delay3/1 -> Add/2
  Delay4/1 -> CwEdMetric/1
